simulink model "example_PV_Inverter"  (R2013b)
settings: Solver=ode45  StartTime=0*24*3600  StopTime=24*3600  MaxStep=60  RelTol=1e-4
libraries: carnot x4
settings Model: Creator=drhf  LastModifiedBy=drhf
settings DataIOCC: SignalLoggingSaveFormat=ModelDataLogs
settings OptimizationCC: ExpressionDepthLimit=2147483647
settings DebuggingCC: FcnCallInpInsideContextMsg=UseLocalSettings  StateNameClashWarn=warning
settings GRTTargetCC: CombineOutputUpdateFcns=off  GRTInterface=on

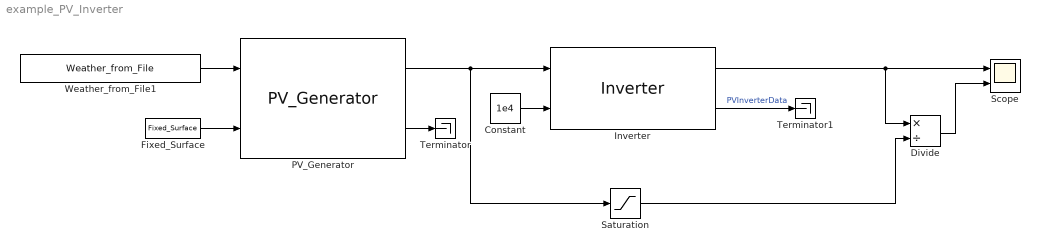
== system example_PV_Inverter ==
  Constant : Constant  Value=1e4
  Divide : Product  Inputs=*/
  Fixed_Surface : carnot/Weather/Fixed_Surface  colangle=30  colazi=0  colrot=0
  Inverter : carnot/Source/Electric_Generator/Inverter  P0=9000  ol=1.2  power_steps=[0 0.05 0.1 0.2 0.3 0.5 1 1.2]  eta_steps=[0 0.924 0.958 0.974 0.979 0.981 0.98 0.95]  standby=0
  PV_Generator : carnot/Source/Electric_Generator/PV_Generator  Wp=10000  delta_Wp_K=0.0047  fgen=0.91 % 0.06 power missmatch, 0.01 diodes, 0.02 data sheet tolerance
  Saturation : Saturate  UpperLimit=inf  LowerLimit=1e-3
  Scope : Scope  NumInputPorts=2
      settings: YMin=-5~-5  YMax=5~5  SaveName=ScopeData2
  Terminator : Terminator
  Terminator1 : Terminator
  Weather_from_File1 : carnot/Weather/Weather_from_File  file=DE_TRY2010_13_averageYear  ext=.mat
  wires:
  PV_Generator/1 -> Inverter/1, Saturation/1
  Inverter/1 -> Scope/1, Divide/1
  Divide/1 -> Scope/2
  Fixed_Surface/1 -> PV_Generator/2
  Weather_from_File1/1 -> PV_Generator/1
  Saturation/1 -> Divide/2
  PV_Generator/2 -> Terminator/1
  Constant/1 -> Inverter/2
  Inverter/2 -> Terminator1/1  "PVInverterData"
